simulink model "em"  (R2023b)
settings: Solver=FixedStepDiscrete  StartTime=0.0  StopTime=3180  FixedStep=0.015  RelTol=1e-3
settings Model: TunableVars=w,V,maxK,lb_mm,ub_mm,epsilon  TunableVarsStorageClass=Auto,Auto,Auto,Auto,Auto,Auto  TunableVarsTypeQualifier=,,,,,  Creator=Inver  LastModifiedBy=Inver
settings DataIOCC: ExternalInput=ds_tm.getElement('rTVS'),ds_tm.getElement('rEQUAL'),ds_tm.getElement('F_raw'),ds_tm.getElement('D_raw')  LoadExternalInput=on
settings OptimizationCC: DefaultParameterBehavior=Inlined  GainParamInheritBuiltInType=on  UseFloatMulNetSlope=on  UseSpecifiedMinMax=on  InlineInvariantSignals=on  StrengthReduction=on  PassReuseOutputArgsAs=Individual arguments  ZeroExternalMemoryAtStartup=off  ZeroInternalMemoryAtStartup=off  NoFixptDivByZeroProtection=on  EfficientFloat2IntCast=on  LifeSpan=1  OptimizeBlockOrder=speed  DifferentSizesBufferReuse=on  OptimizationPriority=Speed  MultiThreadedLoops=on  EfficientTunableParamExpr=on
settings DebuggingCC: ReadBeforeWriteMsg=DisableAll  WriteAfterWriteMsg=DisableAll  WriteAfterReadMsg=DisableAll  MultiTaskDSMMsg=none  ParameterTunabilityLossMsg=error
settings HardwareCC: ProdBitPerPointer=32  ProdBitPerSizeT=32  ProdBitPerPtrDiffT=32  ProdLargestAtomicInteger=Long  ProdLargestAtomicFloat=Double  ProdWordSize=32  ProdLongLongMode=on  ProdHWDeviceType=ARM Compatible->ARM Cortex-M
settings ModelReferenceCC: UpdateModelReferenceTargets=IfOutOfDate
settings SFSimCC: SFSimEcho=off  MATLABDynamicMemAlloc=off
settings RTWCC: Description=Embedded Coder  SystemTargetFile=ert.tlc  GenCodeOnly=on  PackageGeneratedCodeAndArtifacts=on  TemplateMakefile=ert_default_tmf  Toolchain=GNU Tools for ARM Embedded Processors  BuildConfiguration=Faster Runs
settings CodeAppCC: ForceParamTrailComments=on  IgnoreCustomStorageClasses=off  SimulinkDataObjDesc=on  CustomSymbolStrGlobalVar=rt$N$M_em  CustomSymbolStrType=$N$M_em  CustomSymbolStrBlkIO=$N$M  SimulinkBlockComments=off
settings ERTTargetCC: TargetLangStandard=C99 (ISO)  GenerateSampleERTMain=on  CombineSignalStateStructs=on  SuppressErrorStatus=on  CodeInterfacePackaging=Reusable function  SupportNonFinite=off  SupportComplex=off  InlinedParameterPlacement=NonHierarchical  RootIOFormat=Structure reference  ERTCustomFileTemplate=example_file_process.tlc  GlobalDataDefinition=InSeparateSourceFile  DataDefinitionFile=data.c  GlobalDataReference=InSeparateHeaderFile  ERTFilePackagingFormat=CompactWithDataFile  DataReferenceFile=data.h

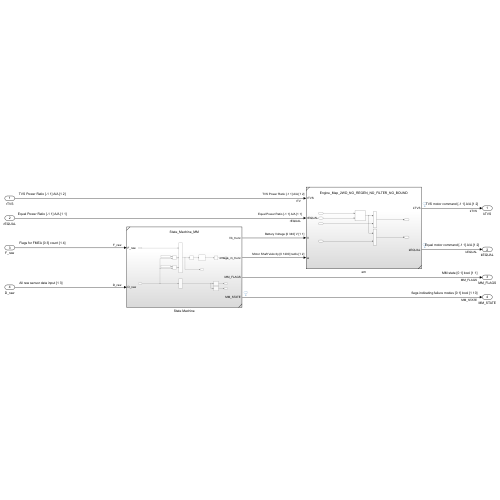
[thumbnail: Simulink's stored preview of the top-level diagram]
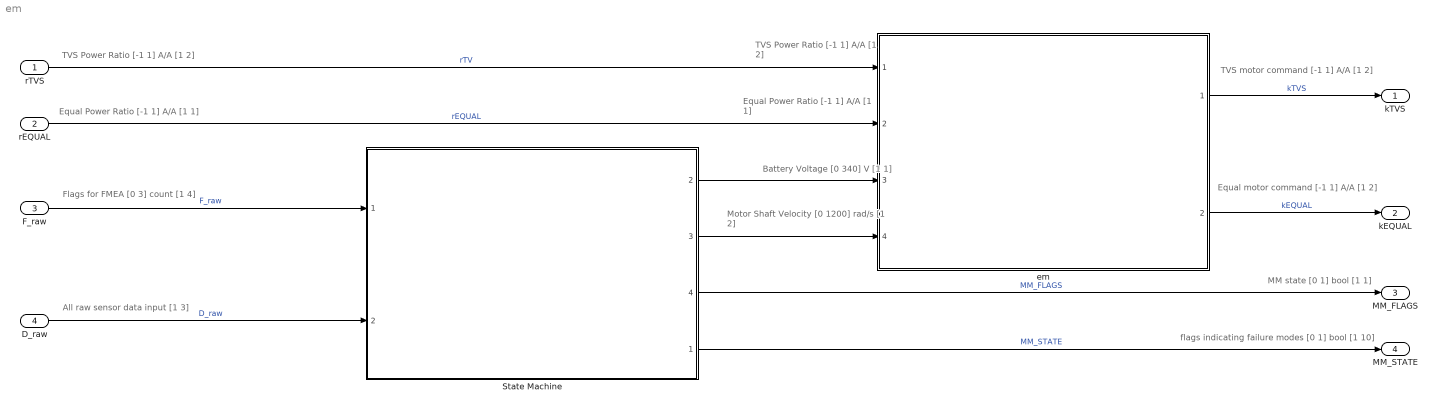
== system em ==
  note: flags indicating failure modes [0 1] bool [1 10]
  note: MM state [0 1] bool [1 1]
  note: Equal motor command [-1 1] A/A [1 2]
  note: TVS motor command [-1 1] A/A [1 2]
  note: TVS Power Ratio [-1 1] A/A [1 2]
  note: Equal Power Ratio [-1 1] A/A [1 1]
  note: All raw sensor data input [1 3]
  note: Flags for FMEA [0 3] count [1 4]
  note: Motor Shaft Velocity [0 1200] rad/s [1 2]
  note: Equal Power Ratio [-1 1] A/A [1 1]
  note: Battery Voltage [0 340] V [1 1]
  note: TVS Power Ratio [-1 1] A/A [1 2]
  rTVS : Inport  PortDimensions=[1 2]
  rEQUAL : Inport  Port=2  PortDimensions=[1 1]
  F_raw : Inport  Port=3  PortDimensions=[1 4]
  D_raw : Inport  Port=4  PortDimensions=[1 3]
  State Machine : Subsystem  ReferencedSubsystem=State_Machine_MM
      settings: PortSchema="{\"entries\":[{\"content\":{\"sides\":[{\"content\":{\"connectorIds\":[\"In1\",\"In2\"]},\"type\":\"ConnectorPlacement.EquallySpacedRectSide\",\"uuid\":\"3ad5cc8f-5c24-495b-b7bf-c12b21ca6743\"},{\"content\":{\"connectorIds\":[\"Out2\",\"Out3\",\"Out4\",\"Out1\"],\"side\":\"RIGHT\"},\"type\":\"ConnectorPlacement.EquallySpacedRectSide\",\"uuid\":\"199951c7-79be-4b7a-80a1-2c2fec8c516f\"},{\"content\":{\"side\":\"TOP\"},\"type\":\"ConnectorPlacement.EquallySpacedRectSide\",\"uuid\":\"296cd14f-6cd9-481e-92b9-c36b65280b3a\"}]},\"type\":\"ConnectorPlacement.EquallySpacedConnector\",\"uuid\":\"592bd7cc-8272-4bf2-9b34-0f5ee02d28bc\"}],\"packageUris\":[\"http://schema.mathworks.com/mf0/Connector/R2020b\"],\"version\":\"1.0\"}"
  em : Subsystem  ReferencedSubsystem=Engine_Map_2WD_NO_REGEN_NO_FILTER_NO_BOUND
  kTVS : Outport
  kEQUAL : Outport  Port=2
  MM_FLAGS : Outport  Port=3
  MM_STATE : Outport  Port=4
  wires:
  em/2 -> kEQUAL/1  "kEQUAL"
  em/1 -> kTVS/1  "kTVS"
  rEQUAL/1 -> em/2  "rEQUAL"
  rTVS/1 -> em/1  "rTV"
  State Machine/2 -> em/3
  State Machine/3 -> em/4
  State Machine/4 -> MM_FLAGS/1  "MM_FLAGS"
  State Machine/1 -> MM_STATE/1  "MM_STATE"
  D_raw/1 -> State Machine/2  "D_raw"
  F_raw/1 -> State Machine/1  "F_raw"
